simulink model "Steady_State_Linear circuit"  (R2023b)
settings: Solver=VariableStepAuto  StartTime=0.0  StopTime=10.0  RelTol=1e-3
libraries: spsACVoltageSourceLib x1, spsSeriesRLCBranchLib x1, spsCurrentMeasurementLib x1, spsACCurrentSourceLib x1, spsImpedanceMeasurementLib x1, spsVoltageMeasurementLib x1, spsParallelRLCBranchLib x1, spspowerguiLib x1
settings Model: Creator=erandum  LastModifiedBy=erandum

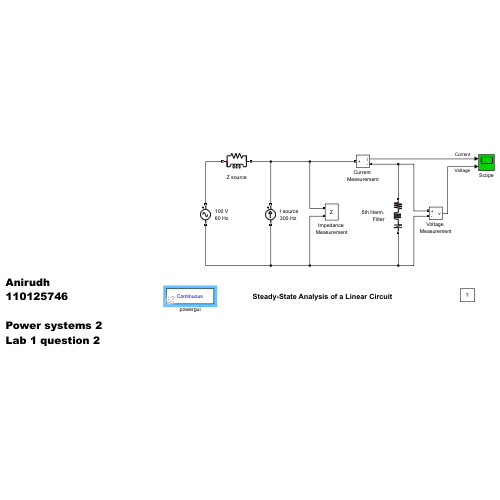
[thumbnail: Simulink's stored preview of the top-level diagram]
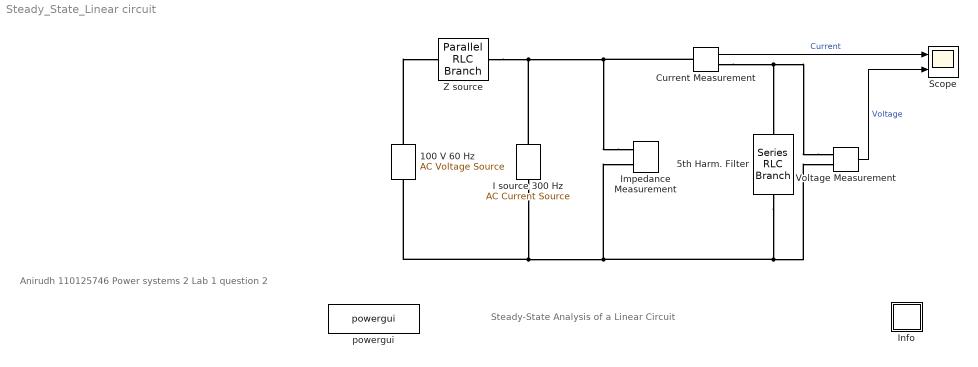
== system Steady_State_Linear circuit ==
  note: Steady-State Analysis of a Linear Circuit
  note: Anirudh
      | 110125746
      |
      | Power systems 2
      | Lab 1 question 2
  100 V 60 Hz : spsACVoltageSourceLib/AC Voltage Source  Description=source block  Amplitude=100  Phase=0  Frequency=60  SampleTime=0  Measurements=None  BusType=swing  Pref=10e3  Qref=0  Qmin=-inf  Qmax=+inf
      settings: AttributesFormatString=\n
  5th Harm. Filter : spsSeriesRLCBranchLib/Series RLC Branch  LConnTagsString=__new0  RConnTagsString=__new0  BranchType=RLC  Resistance=1.27  Inductance=107.42e-03  SetiL0=off  InitialCurrent=0  Capacitance=2.62e-06  Setx0=off  InitialVoltage=0  Measurements=None
  Current Measurement : spsCurrentMeasurementLib/Current Measurement  Tag=PoWeRsYsTeMmEaSuReMeNt  PhasorSimulation=off  OutputType=Magnitude  PSBequivalent=0
      settings: AttributesFormatString=\n
  I source 300 Hz : spsACCurrentSourceLib/AC Current Source  Amplitude=1  Phase=-30  Frequency=300  SampleTime=0  Measurements=None
      settings: AttributesFormatString=\n
  Impedance Measurement : spsImpedanceMeasurementLib/Impedance Measurement  LConnTagsString=+|-  Factor=1
      settings: AttributesFormatString=\n
  Info : Subsystem
      settings: OpenFcn="showExample(\"simscapeelectricalsps/SteadyStateAnalysisExample\")"
      mask Display: disp('?')
  Scope : Scope  NumInputPorts=2
  Voltage Measurement : spsVoltageMeasurementLib/Voltage Measurement  Tag=PoWeRsYsTeMmEaSuReMeNt  PhasorSimulation=off  OutputType=Magnitude  PSBequivalent=0
  Z source : spsParallelRLCBranchLib/Parallel RLC Branch  LConnTagsString=a  RConnTagsString=__new0  BranchType=RL  Resistance=37.7  Inductance=10e-03  SetiL0=off  InitialCurrent=0  Capacitance=0  Setx0=off  InitialVoltage=0  Measurements=None
  powergui : spspowerguiLib/powergui  Priority=2  SimulationMode=Continuous  SampleTime=50e-6  frequency=60  Iterations=50  frequencyindice=60  Pbase=100e6  ErrMax=1e-4  UnitsV=kV  UnitsW=MW  buscounter=0  FunctionMessages=off  echomessages=off  EnableUseOfTLC=off  CurrentSourceSwitches=off  DisableSnubberDevices=off  DisableRonSwitches=off  DisableVfSwitches=off  DisplayEquations=off  AutomaticDiscreteSolvers=off  SolverType=Tustin  Interpol=off  ExternalGateDelay=off  methode=off  Ts=0  x0status=blocks  SPID=off  SwTol=0  HookPort=off  NonlinearTolerance=1e-4  nMaxIteration=100  ContinueOnMaxIteration=off  RestoreLinks=warning  ResistiveCurrentMeasurement=off  Frange=0:2:1000  Ylog=off  Xlog=off  ShowGrid=off  save=off  variable=ZData  structure=0  ZoomFFT=on  StartTime=0.0  cycles=1  DisplayStyle=off  fundamental=60  FreqAxis=off  MaxFrequency=1000  frequencyindicesteady=1  RmsSteady=1  display=off
  wires:
  Current Measurement/1 -> Scope/1  "Current"
  Voltage Measurement/1 -> Scope/2  "Voltage"
  connections:
  100 V 60 Hz/LConn1 -- I source 300 Hz/LConn1 -- Impedance Measurement/LConn2 -- 5th Harm. Filter/RConn1 -- Voltage Measurement/LConn2
  Voltage Measurement/LConn1 -- Current Measurement/RConn1 -- 5th Harm. Filter/LConn1
  Impedance Measurement/LConn1 -- Current Measurement/LConn1 -- I source 300 Hz/RConn1 -- Z source/RConn1
  100 V 60 Hz/RConn1 -- Z source/LConn1

== system Steady_State_Linear circuit/Info ==
